simulink model "finalcode"  (R2020a)
settings: Solver=FixedStepDiscrete  StartTime=0.0  StopTime=1  FixedStep=0.0005  RelTol=1e-3  EnableMultiTasking=on
undefined symbols (not defined in the file): acc_calmax1, acc_calmax2, acc_calmin1, acc_calmin2, akemancanshu, angle_middle, bre, bre_calmax, bre_calmin, chasuniujvvvv_hou, chasuniujvvvv_qian, chasuuuu, ecucoder_acal, I_AN01_5K1, I_AN03_5V, I_AN04_5V, kd, kddd, ki, kiii, kp, kppp, leftmax, O_SW06_HS1A, P11111, P22222, PIDmodel, PPPP, rightmax, slip, slip_big, slip_little, slipmodel, T_add, T_del, tiaoshi, TTTTTyouren, vvvv, zhiling
libraries: ec5744lib x305, canmsglib x97, simulink x23
(part 3 of 11)

== system finalcode/无人TX/Toworkstation/toworkstation/toworkstation ==
  CAN Pack : canmsglib/CAN Pack  CANdbFile=C:\Users\Liu keliang\Desktop\HRT2023\HRT23赛季刘科良\CANdbc\toworkstation.dbc  MsgList=(none)  MsgName=toworkstation  MsgIDType=Standard (11-bit identifier)  MsgIdentifier=562  MsgLength=8  Remote=off  ApplyMinMax=off  BusOutput=off  SignalInfo={'youhou','0','16','LE','signed','Standard','0','1','0','-Inf','Inf';'youqian','16','16','LE','signed','Standard','0','1','0','-Inf','Inf';'zuohou','32','16','LE','signed','Standard','0','1','0','-Inf','Inf';'zuoqian','48','16','LE','signed','Standard','0','1','0','-Inf','Inf'}
      settings: SourceProductBaseCode=ME,XP,VN  DataFormat=CANdb specified signals
  CAN Pack1 : canmsglib/CAN Pack  CANdbFile=C:\Users\86155\Desktop\HRT2024\qkx\can\angle.dbc  MsgList=New_Message_3  MsgName=New_Message_3  MsgIDType=Standard (11-bit identifier)  MsgIdentifier=563  MsgLength=8  Remote=off  ApplyMinMax=off  BusOutput=off  SignalInfo={'actual_speed','48','16','LE','signed','Standard','0','1','0','-Inf','Inf';'bianmaqi','0','16','LE','signed','Standard','0','1','0','-Inf','Inf';'steer','16','16','LE','signed','Standard','0','1','0','-Inf','Inf';'target_speed','32','16','LE','unsigned','Standard','0','1','0','-Inf','Inf'}
      settings: SourceProductBaseCode=ME,XP,VN  DataFormat=CANdb specified signals
  CAN Pack2 : canmsglib/CAN Pack  CANdbFile=C:\Users\86155\Desktop\HRT2024\qkx\can\niujv.dbc  MsgList=New_Message_2  MsgName=New_Message_2  MsgIDType=Standard (11-bit identifier)  MsgIdentifier=561  MsgLength=8  Remote=off  ApplyMinMax=off  BusOutput=off  SignalInfo={'T_youhou','48','16','LE','signed','Standard','0','1','0','-Inf','Inf';'T_youqian','16','16','LE','signed','Standard','0','1','0','-Inf','Inf';'T_zuohou','32','16','LE','signed','Standard','0','1','0','-Inf','Inf';'T_zuoqian','0','16','LE','signed','Standard','0','1','0','-Inf','Inf'}
      settings: SourceProductBaseCode=ME,XP,VN  DataFormat=CANdb specified signals
  CANPackMessage : ec5744lib/RapidECU_U4B/04CANCommunication/CANPackMessage  datalength=8  sampletime=-1
      settings: SourceProductName=ECUCoder for MPC5744
  CANPackMessage1 : ec5744lib/RapidECU_U4B/04CANCommunication/CANPackMessage  datalength=8  sampletime=-1
      settings: SourceProductName=ECUCoder for MPC5744
  CANPackMessage2 : ec5744lib/RapidECU_U4B/04CANCommunication/CANPackMessage  datalength=8  sampletime=-1
      settings: SourceProductName=ECUCoder for MPC5744
  CANTransmit : ec5744lib/RapidECU_U4B/04CANCommunication/CANTransmit  canmodule=2  canbuffer=59  canmessageid=hex2dec('232')  canmessagetype=Standard(11-bit ID)  datalength=8  sampletime=-1
      settings: SourceProductName=ECUCoder for MPC5744
  CANTransmit1 : ec5744lib/RapidECU_U4B/04CANCommunication/CANTransmit  canmodule=2  canbuffer=63  canmessageid=hex2dec('233')  canmessagetype=Standard(11-bit ID)  datalength=8  sampletime=-1
      settings: SourceProductName=ECUCoder for MPC5744
  CANTransmit2 : ec5744lib/RapidECU_U4B/04CANCommunication/CANTransmit  canmodule=2  canbuffer=10  canmessageid=hex2dec('231')  canmessagetype=Standard(11-bit ID)  datalength=8  sampletime=-1
      settings: SourceProductName=ECUCoder for MPC5744
  Data Store Read : DataStoreRead  DataStoreName=er_v_lf
  Data Store Read1 : DataStoreRead  DataStoreName=er_v_rb
  Data Store Read10 : DataStoreRead  DataStoreName=torque_youhou
  Data Store Read11 : DataStoreRead  DataStoreName=energyr_youhou
  Data Store Read12 : DataStoreRead  DataStoreName=torque_zuoqian
  Data Store Read13 : DataStoreRead  DataStoreName=energyr_zuoqian
  Data Store Read14 : DataStoreRead  DataStoreName=workstation_steering
  Data Store Read15 : DataStoreRead  DataStoreName=V_guandao
  Data Store Read2 : DataStoreRead  DataStoreName=er_v_rf
  Data Store Read3 : DataStoreRead  DataStoreName=er_v_lb
  Data Store Read4 : DataStoreRead  DataStoreName=V_workstation
  Data Store Read5 : DataStoreRead  DataStoreName=steere
  Data Store Read6 : DataStoreRead  DataStoreName=torque_zuohou
  Data Store Read7 : DataStoreRead  DataStoreName=energyr_zuohou
  Data Store Read8 : DataStoreRead  DataStoreName=torque_youqian
  Data Store Read9 : DataStoreRead  DataStoreName=energyr_youqian
  Data Type Conversion : DataTypeConversion  OutDataTypeStr=uint8
  Data Type Conversion1 : DataTypeConversion  OutDataTypeStr=uint8
  Data Type Conversion2 : DataTypeConversion  OutDataTypeStr=uint8
  Gain{1..2,4..5} (4 alike) : Gain  Gain=1000
  MATLAB Function : MATLAB Function  TreatAsAtomicUnit=on
  MATLAB Function1 : MATLAB Function  TreatAsAtomicUnit=on
  MATLAB Function2 : MATLAB Function  TreatAsAtomicUnit=on
  MATLAB Function3 : MATLAB Function  TreatAsAtomicUnit=on
  MeaModule : ec5744lib/RapidECU_U4B/07Calibration/MeaModule  signal=T232
      settings: SourceProductName=ECUCoder for MPC5744
  MeaModule1 : ec5744lib/RapidECU_U4B/07Calibration/MeaModule  signal=T233
      settings: SourceProductName=ECUCoder for MPC5744
  Terminator : Terminator
  Terminator1 : Terminator
  Terminator2 : Terminator
  wires:
  CANPackMessage/1 -> Data Type Conversion/1
  CAN Pack/1 -> CANPackMessage/1
  CANTransmit/1 -> MeaModule/1
  MeaModule/1 -> Terminator/1
  Data Type Conversion/1 -> CANTransmit/1
  CANTransmit1/1 -> MeaModule1/1
  MeaModule1/1 -> Terminator1/1
  CANPackMessage1/1 -> Data Type Conversion1/1
  CAN Pack1/1 -> CANPackMessage1/1
  Data Type Conversion1/1 -> CANTransmit1/1
  Data Store Read14/1 -> Gain4/1
  Data Store Read5/1 -> Gain5/1
  Data Store Read1/1 -> CAN Pack/1
  Data Store Read2/1 -> CAN Pack/2
  Data Store Read3/1 -> CAN Pack/3
  Data Store Read/1 -> CAN Pack/4
  CANPackMessage2/1 -> Data Type Conversion2/1
  CANTransmit2/1 -> Terminator2/1
  CAN Pack2/1 -> CANPackMessage2/1
  Data Type Conversion2/1 -> CANTransmit2/1
  Data Store Read12/1 -> MATLAB Function/1(T)
  Data Store Read13/1 -> MATLAB Function/2(NT)
  MATLAB Function/1(y) -> CAN Pack2/4
  Data Store Read6/1 -> MATLAB Function1/1(T)
  Data Store Read7/1 -> MATLAB Function1/2(NT)
  MATLAB Function1/1(y) -> CAN Pack2/3
  Data Store Read8/1 -> MATLAB Function2/1(T)
  Data Store Read9/1 -> MATLAB Function2/2(NT)
  MATLAB Function2/1(y) -> CAN Pack2/2
  Data Store Read10/1 -> MATLAB Function3/1(T)
  Data Store Read11/1 -> MATLAB Function3/2(NT)
  MATLAB Function3/1(y) -> CAN Pack2/1
  Data Store Read4/1 -> Gain1/1
  Gain4/1 -> CAN Pack1/2
  Gain5/1 -> CAN Pack1/3
  Gain1/1 -> CAN Pack1/4
  Gain2/1 -> CAN Pack1/1
  Data Store Read15/1 -> Gain2/1

== system finalcode/Subsystem/Rx/283 285左前/Subsystem1/Subsystem ==
  ID : Inport
  msg : Inport  Port=2
  Enable : EnablePort
  CAN Pack : canmsglib/CAN Pack  Commented=on  CANdbFile=D:\desktop\enable.dbc  MsgList=(none)  MsgName=AMK_ActualValue1  MsgIDType=Standard (11-bit identifier)  MsgIdentifier=643  MsgLength=8  Remote=off  ApplyMinMax=off  BusOutput=off  SignalInfo={'AMK_ActualVelocity','16','16','LE','signed','Standard','0','1','0','0','65535';'AMK_MagnetizingCurrent','48','16','LE','signed','Standard','0','1','0','0','65535';'AMK_TorqueCurrent','32','16','LE','signed','Standard','0','1','0','0','65535';'AMK_bDcOn1','12','1','LE','unsigned','Standard','0','1','0','0','1';'AMK_bDerating1','15','1','LE','unsigned','Standard','0','1','0','0','1';'AMK_bError1','9','1','LE','unsigned','Standard','0','1','0','0','1';'AMK_bInverterOn1','14','1','LE','unsigned','Standard','0','1','0','0','1';'AMK_bQuitDcOn1','11','1','LE','unsigned','Standard','0','1','0','0','1';'AMK_bQuitInverterOn1','13','1','LE','unsigned','Standard','0','1','0','0','1';'AMK_bReserve1','0','8','LE','unsigned','Standard','0','1','0','0','255';'AMK_bSystemReady1','8','1','LE','unsigned','Standard','0','1','0','0','1';'AMK_bWarn1','10','1','LE','unsigned','Standard','0','1','0','0','1'}
      settings: SourceProductBaseCode=ME,XP,VN  DataFormat=CANdb specified signals
  CAN Unpack : canmsglib/CAN Unpack  CANdbFile=C:\Users\86155\Desktop\HRT2024\qkx\can\enable.dbc  MsgList=(none)  MsgName=AMK_ActualValue2  MsgIDType=Standard (11-bit identifier)  MsgIdentifier=645  MsgLength=8  SignalInfo={'AMK_ErrorInfo','32','16','LE','unsigned','Standard','0','1','0','0','65535';'AMK_TempIGBT','48','16','LE','signed','Standard','0','1','0','-32768','32767';'AMK_TempInverter','16','16','LE','signed','Standard','0','1','0','-32768','32767';'AMK_TempMotor','0','16','LE','signed','Standard','0','1','0','-32768','32767'}  IDPort=off  TimestampPort=off  ErrorPort=off  RemotePort=off  LengthPort=off  StatusPort=off  ApplyMinMax=off
      settings: SourceProductBaseCode=ME,XP,VN  DataFormat=CANdb specified signals
  CANPackMessage : ec5744lib/RapidECU_U4B/04CANCommunication/CANPackMessage  Commented=on  datalength=8  sampletime=-1
      settings: SourceProductName=ECUCoder for MPC5744
  CANUnPackMessage : ec5744lib/RapidECU_U4B/04CANCommunication/CANUnPackMessage  datalength=8  canmessagetype=Standard(11-bit ID)  sampletime=-1
      settings: SourceProductName=ECUCoder for MPC5744
  wires:
  msg/1 -> CANUnPackMessage/2
  CANUnPackMessage/1 -> CAN Unpack/1
  ID/1 -> CANUnPackMessage/1
  CANPackMessage/1 -> ?
  CAN Pack/1 -> CANPackMessage/1

== system finalcode/Subsystem/Rx/283 285左前/Subsystem2/Subsystem ==
  ID : Inport
  msg : Inport  Port=2
  Enable : EnablePort
  CAN Pack : canmsglib/CAN Pack  Commented=on  CANdbFile=D:\desktop\enable.dbc  MsgList=(none)  MsgName=AMK_ActualValue1  MsgIDType=Standard (11-bit identifier)  MsgIdentifier=643  MsgLength=8  Remote=off  ApplyMinMax=off  BusOutput=off  SignalInfo={'AMK_ActualVelocity','16','16','LE','signed','Standard','0','1','0','0','65535';'AMK_MagnetizingCurrent','48','16','LE','signed','Standard','0','1','0','0','65535';'AMK_TorqueCurrent','32','16','LE','signed','Standard','0','1','0','0','65535';'AMK_bDcOn1','12','1','LE','unsigned','Standard','0','1','0','0','1';'AMK_bDerating1','15','1','LE','unsigned','Standard','0','1','0','0','1';'AMK_bError1','9','1','LE','unsigned','Standard','0','1','0','0','1';'AMK_bInverterOn1','14','1','LE','unsigned','Standard','0','1','0','0','1';'AMK_bQuitDcOn1','11','1','LE','unsigned','Standard','0','1','0','0','1';'AMK_bQuitInverterOn1','13','1','LE','unsigned','Standard','0','1','0','0','1';'AMK_bReserve1','0','8','LE','unsigned','Standard','0','1','0','0','255';'AMK_bSystemReady1','8','1','LE','unsigned','Standard','0','1','0','0','1';'AMK_bWarn1','10','1','LE','unsigned','Standard','0','1','0','0','1'}
      settings: SourceProductBaseCode=ME,XP,VN  DataFormat=CANdb specified signals
  CAN Unpack : canmsglib/CAN Unpack  CANdbFile=C:\Users\86155\Desktop\HRT2024\qkx\can\enable.dbc  MsgList=(none)  MsgName=AMK_ActualValue1  MsgIDType=Standard (11-bit identifier)  MsgIdentifier=643  MsgLength=8  SignalInfo={'AMK_ActualVelocity','16','16','LE','signed','Standard','0','1','0','-32768','32767';'AMK_MagnetizingCurrent','48','16','LE','signed','Standard','0','1','0','-32768','32767';'AMK_TorqueCurrent','32','16','LE','signed','Standard','0','1','0','-32768','32767';'AMK_bDcOn1','12','1','LE','unsigned','Standard','0','1','0','0','1';'AMK_bDerating1','15','1','LE','unsigned','Standard','0','1','0','0','1';'AMK_bError1','9','1','LE','unsigned','Standard','0','1','0','0','1';'AMK_bInverterOn1','14','1','LE','unsigned','Standard','0','1','0','0','1';'AMK_bQuitDcOn1','11','1','LE','unsigned','Standard','0','1','0','0','1';'AMK_bQuitInverterOn1','13','1','LE','unsigned','Standard','0','1','0','0','1';'AMK_bReserve1','0','8','LE','unsigned','Standard','0','1','0','0','255';'AMK_bSystemReady1','8','1','LE','unsigned','Standard','0','1','0','0','1';'AMK_bWarn1','10','1','LE','unsigned','Standard','0','1','0','0','1'}  IDPort=off  TimestampPort=off  ErrorPort=off  RemotePort=off  LengthPort=off  StatusPort=off  ApplyMinMax=off
      settings: SourceProductBaseCode=ME,XP,VN  DataFormat=CANdb specified signals
  CANPackMessage : ec5744lib/RapidECU_U4B/04CANCommunication/CANPackMessage  Commented=on  datalength=8  sampletime=-1
      settings: SourceProductName=ECUCoder for MPC5744
  CANUnPackMessage : ec5744lib/RapidECU_U4B/04CANCommunication/CANUnPackMessage  datalength=8  canmessagetype=Standard(11-bit ID)  sampletime=-1
      settings: SourceProductName=ECUCoder for MPC5744
  Data Store Write : DataStoreWrite  DataStoreName=dianji_velcoity_zuoqian
  Data Store Write1 : DataStoreWrite  DataStoreName=er_v_lf
  Data Store Write2 : DataStoreWrite  DataStoreName=er_T_lf
  MATLAB Function : MATLAB Function  TreatAsAtomicUnit=on
  MeaModule : ec5744lib/RapidECU_U4B/07Calibration/MeaModule  signal=v_zuoqian
      settings: SourceProductName=ECUCoder for MPC5744
  wires:
  msg/1 -> CANUnPackMessage/2
  CANUnPackMessage/1 -> CAN Unpack/1
  ID/1 -> CANUnPackMessage/1
  CANPackMessage/1 -> ?
  CAN Unpack/1 -> Data Store Write1/1, MATLAB Function/1(u)
  MATLAB Function/1(y) -> MeaModule/1
  CAN Unpack/2 -> CAN Pack/2
  CAN Unpack/4 -> CAN Pack/5
  CAN Unpack/6 -> CAN Pack/8
  CAN Unpack/8 -> CAN Pack/11
  CAN Unpack/3 -> Data Store Write2/1
  MeaModule/1 -> Data Store Write/1

== system finalcode/Subsystem/Rx/284 286右前/Subsystem1/Subsystem ==
  ID : Inport
  msg : Inport  Port=2
  Enable : EnablePort
  CAN Pack : canmsglib/CAN Pack  Commented=on  CANdbFile=D:\desktop\enable.dbc  MsgList=(none)  MsgName=AMK_ActualValue1  MsgIDType=Standard (11-bit identifier)  MsgIdentifier=643  MsgLength=8  Remote=off  ApplyMinMax=off  BusOutput=off  SignalInfo={'AMK_ActualVelocity','16','16','LE','signed','Standard','0','1','0','0','65535';'AMK_MagnetizingCurrent','48','16','LE','signed','Standard','0','1','0','0','65535';'AMK_TorqueCurrent','32','16','LE','signed','Standard','0','1','0','0','65535';'AMK_bDcOn1','12','1','LE','unsigned','Standard','0','1','0','0','1';'AMK_bDerating1','15','1','LE','unsigned','Standard','0','1','0','0','1';'AMK_bError1','9','1','LE','unsigned','Standard','0','1','0','0','1';'AMK_bInverterOn1','14','1','LE','unsigned','Standard','0','1','0','0','1';'AMK_bQuitDcOn1','11','1','LE','unsigned','Standard','0','1','0','0','1';'AMK_bQuitInverterOn1','13','1','LE','unsigned','Standard','0','1','0','0','1';'AMK_bReserve1','0','8','LE','unsigned','Standard','0','1','0','0','255';'AMK_bSystemReady1','8','1','LE','unsigned','Standard','0','1','0','0','1';'AMK_bWarn1','10','1','LE','unsigned','Standard','0','1','0','0','1'}
      settings: SourceProductBaseCode=ME,XP,VN  DataFormat=CANdb specified signals
  CAN Unpack : canmsglib/CAN Unpack  CANdbFile=C:\Users\86155\Desktop\HRT2024\qkx\can\enable_youqian.dbc  MsgList=AMK_ActualValue2  MsgName=AMK_ActualValue2  MsgIDType=Standard (11-bit identifier)  MsgIdentifier=646  MsgLength=8  SignalInfo={'AMK_ErrorInfo','32','16','LE','unsigned','Standard','0','1','0','0','65535';'AMK_TempIGBT','48','16','LE','signed','Standard','0','1','0','-32768','32767';'AMK_TempInverter','16','16','LE','signed','Standard','0','1','0','-32768','32767';'AMK_TempMotor','0','16','LE','signed','Standard','0','1','0','-32768','32767'}  IDPort=off  TimestampPort=off  ErrorPort=off  RemotePort=off  LengthPort=off  StatusPort=off  ApplyMinMax=off
      settings: SourceProductBaseCode=ME,XP,VN  DataFormat=CANdb specified signals
  CANPackMessage : ec5744lib/RapidECU_U4B/04CANCommunication/CANPackMessage  Commented=on  datalength=8  sampletime=-1
      settings: SourceProductName=ECUCoder for MPC5744
  CANUnPackMessage : ec5744lib/RapidECU_U4B/04CANCommunication/CANUnPackMessage  datalength=8  canmessagetype=Standard(11-bit ID)  sampletime=-1
      settings: SourceProductName=ECUCoder for MPC5744
  wires:
  msg/1 -> CANUnPackMessage/2
  CANUnPackMessage/1 -> CAN Unpack/1
  ID/1 -> CANUnPackMessage/1
  CANPackMessage/1 -> ?
  CAN Pack/1 -> CANPackMessage/1

== system finalcode/Subsystem/Rx/284 286右前/Subsystem2/Subsystem ==
  ID : Inport
  msg : Inport  Port=2
  Enable : EnablePort
  CAN Pack : canmsglib/CAN Pack  Commented=on  CANdbFile=D:\desktop\enable.dbc  MsgList=(none)  MsgName=AMK_ActualValue1  MsgIDType=Standard (11-bit identifier)  MsgIdentifier=643  MsgLength=8  Remote=off  ApplyMinMax=off  BusOutput=off  SignalInfo={'AMK_ActualVelocity','16','16','LE','signed','Standard','0','1','0','0','65535';'AMK_MagnetizingCurrent','48','16','LE','signed','Standard','0','1','0','0','65535';'AMK_TorqueCurrent','32','16','LE','signed','Standard','0','1','0','0','65535';'AMK_bDcOn1','12','1','LE','unsigned','Standard','0','1','0','0','1';'AMK_bDerating1','15','1','LE','unsigned','Standard','0','1','0','0','1';'AMK_bError1','9','1','LE','unsigned','Standard','0','1','0','0','1';'AMK_bInverterOn1','14','1','LE','unsigned','Standard','0','1','0','0','1';'AMK_bQuitDcOn1','11','1','LE','unsigned','Standard','0','1','0','0','1';'AMK_bQuitInverterOn1','13','1','LE','unsigned','Standard','0','1','0','0','1';'AMK_bReserve1','0','8','LE','unsigned','Standard','0','1','0','0','255';'AMK_bSystemReady1','8','1','LE','unsigned','Standard','0','1','0','0','1';'AMK_bWarn1','10','1','LE','unsigned','Standard','0','1','0','0','1'}
      settings: SourceProductBaseCode=ME,XP,VN  DataFormat=CANdb specified signals
  CAN Unpack : canmsglib/CAN Unpack  CANdbFile=C:\Users\86155\Desktop\HRT2024\qkx\can\enable_youqian.dbc  MsgList=AMK_ActualValue1  MsgName=AMK_ActualValue1  MsgIDType=Standard (11-bit identifier)  MsgIdentifier=644  MsgLength=8  SignalInfo={'AMK_ActualVelocity','16','16','LE','signed','Standard','0','1','0','-32768','32767';'AMK_MagnetizingCurrent','48','16','LE','signed','Standard','0','1','0','-32768','32767';'AMK_TorqueCurrent','32','16','LE','signed','Standard','0','1','0','-32768','32767';'AMK_bDcOn1','12','1','LE','unsigned','Standard','0','1','0','0','1';'AMK_bDerating1','15','1','LE','unsigned','Standard','0','1','0','0','1';'AMK_bError1','9','1','LE','unsigned','Standard','0','1','0','0','1';'AMK_bInverterOn1','14','1','LE','unsigned','Standard','0','1','0','0','1';'AMK_bQuitDcOn1','11','1','LE','unsigned','Standard','0','1','0','0','1';'AMK_bQuitInverterOn1','13','1','LE','unsigned','Standard','0','1','0','0','1';'AMK_bReserve1','0','8','LE','unsigned','Standard','0','1','0','0','255';'AMK_bSystemReady1','8','1','LE','unsigned','Standard','0','1','0','0','1';'AMK_bWarn1','10','1','LE','unsigned','Standard','0','1','0','0','1'}  IDPort=off  TimestampPort=off  ErrorPort=off  RemotePort=off  LengthPort=off  StatusPort=off  ApplyMinMax=off
      settings: SourceProductBaseCode=ME,XP,VN  DataFormat=CANdb specified signals
  CANPackMessage : ec5744lib/RapidECU_U4B/04CANCommunication/CANPackMessage  Commented=on  datalength=8  sampletime=-1
      settings: SourceProductName=ECUCoder for MPC5744
  CANUnPackMessage : ec5744lib/RapidECU_U4B/04CANCommunication/CANUnPackMessage  datalength=8  canmessagetype=Standard(11-bit ID)  sampletime=-1
      settings: SourceProductName=ECUCoder for MPC5744
  Data Store Write : DataStoreWrite  DataStoreName=dianji_velcoity_youqian
  Data Store Write1 : DataStoreWrite  DataStoreName=er_v_rf
  Data Store Write2 : DataStoreWrite  DataStoreName=er_T_rf
  MATLAB Function : MATLAB Function  TreatAsAtomicUnit=on
  MeaModule : ec5744lib/RapidECU_U4B/07Calibration/MeaModule  signal=v_youqian
      settings: SourceProductName=ECUCoder for MPC5744
  wires:
  msg/1 -> CANUnPackMessage/2
  CANUnPackMessage/1 -> CAN Unpack/1
  ID/1 -> CANUnPackMessage/1
  CANPackMessage/1 -> ?
  CAN Pack/1 -> CANPackMessage/1
  CAN Unpack/1 -> Data Store Write1/1, MATLAB Function/1(u)
  MATLAB Function/1(y) -> MeaModule/1
  CAN Unpack/3 -> Data Store Write2/1
  MeaModule/1 -> Data Store Write/1

== system finalcode/Subsystem/Rx/287 289右后/Subsystem1/Subsystem ==
  ID : Inport
  msg : Inport  Port=2
  Enable : EnablePort
  CAN Pack : canmsglib/CAN Pack  Commented=on  CANdbFile=D:\desktop\enable.dbc  MsgList=(none)  MsgName=AMK_ActualValue1  MsgIDType=Standard (11-bit identifier)  MsgIdentifier=643  MsgLength=8  Remote=off  ApplyMinMax=off  BusOutput=off  SignalInfo={'AMK_ActualVelocity','16','16','LE','signed','Standard','0','1','0','0','65535';'AMK_MagnetizingCurrent','48','16','LE','signed','Standard','0','1','0','0','65535';'AMK_TorqueCurrent','32','16','LE','signed','Standard','0','1','0','0','65535';'AMK_bDcOn1','12','1','LE','unsigned','Standard','0','1','0','0','1';'AMK_bDerating1','15','1','LE','unsigned','Standard','0','1','0','0','1';'AMK_bError1','9','1','LE','unsigned','Standard','0','1','0','0','1';'AMK_bInverterOn1','14','1','LE','unsigned','Standard','0','1','0','0','1';'AMK_bQuitDcOn1','11','1','LE','unsigned','Standard','0','1','0','0','1';'AMK_bQuitInverterOn1','13','1','LE','unsigned','Standard','0','1','0','0','1';'AMK_bReserve1','0','8','LE','unsigned','Standard','0','1','0','0','255';'AMK_bSystemReady1','8','1','LE','unsigned','Standard','0','1','0','0','1';'AMK_bWarn1','10','1','LE','unsigned','Standard','0','1','0','0','1'}
      settings: SourceProductBaseCode=ME,XP,VN  DataFormat=CANdb specified signals
  CAN Unpack : canmsglib/CAN Unpack  CANdbFile=C:\Users\86155\Desktop\HRT2024\qkx\can\enable_youhou.dbc  MsgList=AMK_ActualValue2  MsgName=AMK_ActualValue2  MsgIDType=Standard (11-bit identifier)  MsgIdentifier=649  MsgLength=8  SignalInfo={'AMK_ErrorInfo','32','16','LE','unsigned','Standard','0','1','0','0','65535';'AMK_TempIGBT','48','16','LE','signed','Standard','0','1','0','-32768','32767';'AMK_TempInverter','16','16','LE','signed','Standard','0','1','0','-32768','32767';'AMK_TempMotor','0','16','LE','signed','Standard','0','1','0','-32768','32767'}  IDPort=off  TimestampPort=off  ErrorPort=off  RemotePort=off  LengthPort=off  StatusPort=off  ApplyMinMax=off
      settings: SourceProductBaseCode=ME,XP,VN  DataFormat=CANdb specified signals
  CANPackMessage : ec5744lib/RapidECU_U4B/04CANCommunication/CANPackMessage  Commented=on  datalength=8  sampletime=-1
      settings: SourceProductName=ECUCoder for MPC5744
  CANUnPackMessage : ec5744lib/RapidECU_U4B/04CANCommunication/CANUnPackMessage  datalength=8  canmessagetype=Standard(11-bit ID)  sampletime=-1
      settings: SourceProductName=ECUCoder for MPC5744
  wires:
  msg/1 -> CANUnPackMessage/2
  CANUnPackMessage/1 -> CAN Unpack/1
  ID/1 -> CANUnPackMessage/1
  CANPackMessage/1 -> ?
  CAN Pack/1 -> CANPackMessage/1

== system finalcode/Subsystem/Rx/287 289右后/Subsystem3/Subsystem ==
  ID : Inport
  msg : Inport  Port=2
  Enable : EnablePort
  CAN Pack : canmsglib/CAN Pack  Commented=on  CANdbFile=D:\desktop\enable.dbc  MsgList=(none)  MsgName=AMK_ActualValue1  MsgIDType=Standard (11-bit identifier)  MsgIdentifier=643  MsgLength=8  Remote=off  ApplyMinMax=off  BusOutput=off  SignalInfo={'AMK_ActualVelocity','16','16','LE','signed','Standard','0','1','0','0','65535';'AMK_MagnetizingCurrent','48','16','LE','signed','Standard','0','1','0','0','65535';'AMK_TorqueCurrent','32','16','LE','signed','Standard','0','1','0','0','65535';'AMK_bDcOn1','12','1','LE','unsigned','Standard','0','1','0','0','1';'AMK_bDerating1','15','1','LE','unsigned','Standard','0','1','0','0','1';'AMK_bError1','9','1','LE','unsigned','Standard','0','1','0','0','1';'AMK_bInverterOn1','14','1','LE','unsigned','Standard','0','1','0','0','1';'AMK_bQuitDcOn1','11','1','LE','unsigned','Standard','0','1','0','0','1';'AMK_bQuitInverterOn1','13','1','LE','unsigned','Standard','0','1','0','0','1';'AMK_bReserve1','0','8','LE','unsigned','Standard','0','1','0','0','255';'AMK_bSystemReady1','8','1','LE','unsigned','Standard','0','1','0','0','1';'AMK_bWarn1','10','1','LE','unsigned','Standard','0','1','0','0','1'}
      settings: SourceProductBaseCode=ME,XP,VN  DataFormat=CANdb specified signals
  CAN Unpack : canmsglib/CAN Unpack  CANdbFile=C:\Users\86155\Desktop\HRT2024\qkx\can\enable_youhou.dbc  MsgList=AMK_ActualValue1  MsgName=AMK_ActualValue1  MsgIDType=Standard (11-bit identifier)  MsgIdentifier=647  MsgLength=8  SignalInfo={'AMK_ActualVelocity','16','16','LE','signed','Standard','0','1','0','-32768','32767';'AMK_MagnetizingCurrent','48','16','LE','signed','Standard','0','1','0','-32768','32767';'AMK_TorqueCurrent','32','16','LE','signed','Standard','0','1','0','-32768','32767';'AMK_bDcOn1','12','1','LE','unsigned','Standard','0','1','0','0','1';'AMK_bDerating1','15','1','LE','unsigned','Standard','0','1','0','0','1';'AMK_bError1','9','1','LE','unsigned','Standard','0','1','0','0','1';'AMK_bInverterOn1','14','1','LE','unsigned','Standard','0','1','0','0','1';'AMK_bQuitDcOn1','11','1','LE','unsigned','Standard','0','1','0','0','1';'AMK_bQuitInverterOn1','13','1','LE','unsigned','Standard','0','1','0','0','1';'AMK_bReserve1','0','8','LE','unsigned','Standard','0','1','0','0','255';'AMK_bSystemReady1','8','1','LE','unsigned','Standard','0','1','0','0','1';'AMK_bWarn1','10','1','LE','unsigned','Standard','0','1','0','0','1'}  IDPort=off  TimestampPort=off  ErrorPort=off  RemotePort=off  LengthPort=off  StatusPort=off  ApplyMinMax=off
      settings: SourceProductBaseCode=ME,XP,VN  DataFormat=CANdb specified signals
  CANPackMessage : ec5744lib/RapidECU_U4B/04CANCommunication/CANPackMessage  Commented=on  datalength=8  sampletime=-1
      settings: SourceProductName=ECUCoder for MPC5744
  CANUnPackMessage : ec5744lib/RapidECU_U4B/04CANCommunication/CANUnPackMessage  datalength=8  canmessagetype=Standard(11-bit ID)  sampletime=-1
      settings: SourceProductName=ECUCoder for MPC5744
  Data Store Write : DataStoreWrite  DataStoreName=dianji_velcoity_youhou
  Data Store Write1 : DataStoreWrite  DataStoreName=er_v_rb
  Data Store Write2 : DataStoreWrite  DataStoreName=er_T_rb
  MATLAB Function : MATLAB Function  TreatAsAtomicUnit=on
  MeaModule : ec5744lib/RapidECU_U4B/07Calibration/MeaModule  signal=v_youhou
      settings: SourceProductName=ECUCoder for MPC5744
  wires:
  msg/1 -> CANUnPackMessage/2
  CANUnPackMessage/1 -> CAN Unpack/1
  ID/1 -> CANUnPackMessage/1
  CANPackMessage/1 -> ?
  CAN Pack/1 -> CANPackMessage/1
  MATLAB Function/1(y) -> MeaModule/1
  CAN Unpack/1 -> Data Store Write1/1, MATLAB Function/1(u)
  CAN Unpack/3 -> Data Store Write2/1
  MeaModule/1 -> Data Store Write/1

== system finalcode/Subsystem/Rx/288 290左后/Subsystem1/Subsystem ==
  ID : Inport
  msg : Inport  Port=2
  Enable : EnablePort
  CAN Pack : canmsglib/CAN Pack  Commented=on  CANdbFile=D:\desktop\enable.dbc  MsgList=(none)  MsgName=AMK_ActualValue1  MsgIDType=Standard (11-bit identifier)  MsgIdentifier=643  MsgLength=8  Remote=off  ApplyMinMax=off  BusOutput=off  SignalInfo={'AMK_ActualVelocity','16','16','LE','signed','Standard','0','1','0','0','65535';'AMK_MagnetizingCurrent','48','16','LE','signed','Standard','0','1','0','0','65535';'AMK_TorqueCurrent','32','16','LE','signed','Standard','0','1','0','0','65535';'AMK_bDcOn1','12','1','LE','unsigned','Standard','0','1','0','0','1';'AMK_bDerating1','15','1','LE','unsigned','Standard','0','1','0','0','1';'AMK_bError1','9','1','LE','unsigned','Standard','0','1','0','0','1';'AMK_bInverterOn1','14','1','LE','unsigned','Standard','0','1','0','0','1';'AMK_bQuitDcOn1','11','1','LE','unsigned','Standard','0','1','0','0','1';'AMK_bQuitInverterOn1','13','1','LE','unsigned','Standard','0','1','0','0','1';'AMK_bReserve1','0','8','LE','unsigned','Standard','0','1','0','0','255';'AMK_bSystemReady1','8','1','LE','unsigned','Standard','0','1','0','0','1';'AMK_bWarn1','10','1','LE','unsigned','Standard','0','1','0','0','1'}
      settings: SourceProductBaseCode=ME,XP,VN  DataFormat=CANdb specified signals
  CAN Unpack : canmsglib/CAN Unpack  CANdbFile=C:\Users\86155\Desktop\HRT2024\qkx\can\enabe_zuohou.dbc  MsgList=AMK_ActualValue2  MsgName=AMK_ActualValue2  MsgIDType=Standard (11-bit identifier)  MsgIdentifier=656  MsgLength=8  SignalInfo={'AMK_ErrorInfo','32','16','LE','unsigned','Standard','0','1','0','0','65535';'AMK_TempIGBT','48','16','LE','signed','Standard','0','1','0','-32768','32767';'AMK_TempInverter','16','16','LE','signed','Standard','0','1','0','-32768','32767';'AMK_TempMotor','0','16','LE','signed','Standard','0','1','0','-32768','32767'}  IDPort=off  TimestampPort=off  ErrorPort=off  RemotePort=off  LengthPort=off  StatusPort=off  ApplyMinMax=off
      settings: SourceProductBaseCode=ME,XP,VN  DataFormat=CANdb specified signals
  CANPackMessage : ec5744lib/RapidECU_U4B/04CANCommunication/CANPackMessage  Commented=on  datalength=8  sampletime=-1
      settings: SourceProductName=ECUCoder for MPC5744
  CANUnPackMessage : ec5744lib/RapidECU_U4B/04CANCommunication/CANUnPackMessage  datalength=8  canmessagetype=Standard(11-bit ID)  sampletime=-1
      settings: SourceProductName=ECUCoder for MPC5744
  wires:
  msg/1 -> CANUnPackMessage/2
  CANUnPackMessage/1 -> CAN Unpack/1
  ID/1 -> CANUnPackMessage/1
  CANPackMessage/1 -> ?
  CAN Pack/1 -> CANPackMessage/1

== system finalcode/Subsystem/Rx/288 290左后/Subsystem2/Subsystem ==
  ID : Inport
  msg : Inport  Port=2
  Enable : EnablePort
  CAN Pack : canmsglib/CAN Pack  Commented=on  CANdbFile=D:\desktop\enable.dbc  MsgList=(none)  MsgName=AMK_ActualValue1  MsgIDType=Standard (11-bit identifier)  MsgIdentifier=643  MsgLength=8  Remote=off  ApplyMinMax=off  BusOutput=off  SignalInfo={'AMK_ActualVelocity','16','16','LE','signed','Standard','0','1','0','0','65535';'AMK_MagnetizingCurrent','48','16','LE','signed','Standard','0','1','0','0','65535';'AMK_TorqueCurrent','32','16','LE','signed','Standard','0','1','0','0','65535';'AMK_bDcOn1','12','1','LE','unsigned','Standard','0','1','0','0','1';'AMK_bDerating1','15','1','LE','unsigned','Standard','0','1','0','0','1';'AMK_bError1','9','1','LE','unsigned','Standard','0','1','0','0','1';'AMK_bInverterOn1','14','1','LE','unsigned','Standard','0','1','0','0','1';'AMK_bQuitDcOn1','11','1','LE','unsigned','Standard','0','1','0','0','1';'AMK_bQuitInverterOn1','13','1','LE','unsigned','Standard','0','1','0','0','1';'AMK_bReserve1','0','8','LE','unsigned','Standard','0','1','0','0','255';'AMK_bSystemReady1','8','1','LE','unsigned','Standard','0','1','0','0','1';'AMK_bWarn1','10','1','LE','unsigned','Standard','0','1','0','0','1'}
      settings: SourceProductBaseCode=ME,XP,VN  DataFormat=CANdb specified signals
  CAN Unpack : canmsglib/CAN Unpack  CANdbFile=C:\Users\86155\Desktop\HRT2024\qkx\can\enabe_zuohou.dbc  MsgList=AMK_ActualValue1  MsgName=AMK_ActualValue1  MsgIDType=Standard (11-bit identifier)  MsgIdentifier=648  MsgLength=8  SignalInfo={'AMK_ActualVelocity','16','16','LE','signed','Standard','0','1','0','-32768','32767';'AMK_MagnetizingCurrent','48','16','LE','signed','Standard','0','1','0','-32768','32767';'AMK_TorqueCurrent','32','16','LE','signed','Standard','0','1','0','-32768','32767';'AMK_bDcOn1','12','1','LE','unsigned','Standard','0','1','0','0','1';'AMK_bDerating1','15','1','LE','unsigned','Standard','0','1','0','0','1';'AMK_bError1','9','1','LE','unsigned','Standard','0','1','0','0','1';'AMK_bInverterOn1','14','1','LE','unsigned','Standard','0','1','0','0','1';'AMK_bQuitDcOn1','11','1','LE','unsigned','Standard','0','1','0','0','1';'AMK_bQuitInverterOn1','13','1','LE','unsigned','Standard','0','1','0','0','1';'AMK_bReserve1','0','8','LE','unsigned','Standard','0','1','0','0','255';'AMK_bSystemReady1','8','1','LE','unsigned','Standard','0','1','0','0','1';'AMK_bWarn1','10','1','LE','unsigned','Standard','0','1','0','0','1'}  IDPort=off  TimestampPort=off  ErrorPort=off  RemotePort=off  LengthPort=off  StatusPort=off  ApplyMinMax=off
      settings: SourceProductBaseCode=ME,XP,VN  DataFormat=CANdb specified signals
  CANPackMessage : ec5744lib/RapidECU_U4B/04CANCommunication/CANPackMessage  Commented=on  datalength=8  sampletime=-1
      settings: SourceProductName=ECUCoder for MPC5744
  CANUnPackMessage : ec5744lib/RapidECU_U4B/04CANCommunication/CANUnPackMessage  datalength=8  canmessagetype=Standard(11-bit ID)  sampletime=-1
      settings: SourceProductName=ECUCoder for MPC5744
  Data Store Write : DataStoreWrite  DataStoreName=dianji_velcoity_zuohou
  Data Store Write1 : DataStoreWrite  DataStoreName=er_v_lb
  Data Store Write2 : DataStoreWrite  DataStoreName=er_T_lb
  MATLAB Function : MATLAB Function  TreatAsAtomicUnit=on
  MeaModule : ec5744lib/RapidECU_U4B/07Calibration/MeaModule  signal=v_zuohou
      settings: SourceProductName=ECUCoder for MPC5744
  wires:
  msg/1 -> CANUnPackMessage/2
  CANUnPackMessage/1 -> CAN Unpack/1
  ID/1 -> CANUnPackMessage/1
  CANPackMessage/1 -> ?
  CAN Pack/1 -> CANPackMessage/1
  CAN Unpack/1 -> Data Store Write1/1, MATLAB Function/1(u)
  CAN Unpack/3 -> Data Store Write2/1
  MATLAB Function/1(y) -> MeaModule/1
  MeaModule/1 -> Data Store Write/1
  CAN Unpack/2 -> CAN Pack/2
  CAN Unpack/4 -> CAN Pack/6
  CAN Unpack/5 -> CAN Pack/8
  CAN Unpack/6 -> CAN Pack/10
  CAN Unpack/7 -> CAN Pack/12

== system finalcode/Subsystem/Rx/ebs/Subsystem3/Subsystem ==
  ID : Inport
  msg : Inport  Port=2
  Enable : EnablePort
  CAN Pack : canmsglib/CAN Pack  Commented=on  CANdbFile=C:\Users\Liu keliang\Desktop\HRT2023\HRT23赛季刘科良\CANdbc\workstation.dbc  MsgList=(none)  MsgName=workstation  MsgIDType=Standard (11-bit identifier)  MsgIdentifier=32  MsgLength=5  Remote=off  ApplyMinMax=off  BusOutput=off  SignalInfo={'V','8','8','LE','unsigned','Standard','0','1','0','0','255';'V_Copy_1','16','8','LE','unsigned','Standard','0','1','0','0','255';'controlstart','4','1','LE','unsigned','Standard','0','1','0','-Inf','Inf';'status','0','4','LE','unsigned','Standard','0','1','0','0','15';'steering','24','8','LE','signed','Standard','0','1','0','-128','127';'steering_Copy_1','32','8','LE','signed','Standard','0','1','0','-128','127';'vfeedbackk','40','8','LE','unsigned','Standard','0','1','0','-Inf','Inf'}
      settings: SourceProductBaseCode=ME,XP,VN  DataFormat=CANdb specified signals
  CAN Unpack : canmsglib/CAN Unpack  CANdbFile=C:\Users\Liu keliang\Desktop\HRT2023\HRT23赛季刘科良\CANdbc\ebs.dbc  MsgList=(none)  MsgName=New_Message_1  MsgIDType=Standard (11-bit identifier)  MsgIdentifier=1026  MsgLength=8  SignalInfo={'youhou','48','16','LE','unsigned','Standard','0','1','0','-Inf','Inf';'youqian','16','16','LE','unsigned','Standard','0','1','0','-Inf','Inf';'zuohou','32','16','LE','unsigned','Standard','0','1','0','-Inf','Inf';'zuoqian','0','16','LE','unsigned','Standard','0','1','0','-Inf','Inf'}  IDPort=off  TimestampPort=off  ErrorPort=off  RemotePort=off  LengthPort=off  StatusPort=off  ApplyMinMax=off
      settings: SourceProductBaseCode=ME,XP,VN  DataFormat=CANdb specified signals
  CANPackMessage : ec5744lib/RapidECU_U4B/04CANCommunication/CANPackMessage  Commented=on  datalength=8  sampletime=-1
      settings: SourceProductName=ECUCoder for MPC5744
  CANUnPackMessage : ec5744lib/RapidECU_U4B/04CANCommunication/CANUnPackMessage  datalength=8  canmessagetype=Standard(11-bit ID)  sampletime=-1
      settings: SourceProductName=ECUCoder for MPC5744
  Data Store Write : DataStoreWrite  DataStoreName=oilyouhou
  Data Store Write1 : DataStoreWrite  DataStoreName=oilyouqian
  Data Store Write2 : DataStoreWrite  DataStoreName=oilzuohou
  Data Store Write3 : DataStoreWrite  DataStoreName=oilzuoqian
  wires:
  msg/1 -> CANUnPackMessage/2
  CANUnPackMessage/1 -> CAN Unpack/1
  ID/1 -> CANUnPackMessage/1
  CANPackMessage/1 -> ?
  CAN Pack/1 -> CANPackMessage/1
  CAN Unpack/2 -> Data Store Write1/1
  CAN Unpack/1 -> Data Store Write/1
  CAN Unpack/3 -> Data Store Write2/1
  CAN Unpack/4 -> Data Store Write3/1

== system finalcode/Subsystem/Rx/lcu——receive/Subsystem1/Subsystem ==
  ID : Inport
  msg : Inport  Port=2
  Enable : EnablePort
  CAN Pack : canmsglib/CAN Pack  Commented=on  CANdbFile=C:\Users\Liu keliang\Desktop\HRT2023\HRT23赛季刘科良\CANdbc\enzbled.dbc  MsgList=(none)  MsgName=ecu156  MsgIDType=Standard (11-bit identifier)  MsgIdentifier=342  MsgLength=8  Remote=off  ApplyMinMax=off  BusOutput=off  SignalInfo={'ASMS','3','1','LE','unsigned','Standard','0','1','0','-Inf','Inf';'enable','32','8','LE','unsigned','Standard','0','1','0','0','255';'error','16','8','LE','unsigned','Standard','0','1','0','0','255';'match_model','8','4','LE','unsigned','Standard','0','1','0','0','15';'matchmodel_shucai','24','3','LE','unsigned','Standard','0','1','0','0','6';'model_confirm','27','1','LE','unsigned','Standard','0','1','0','0','1';'res','40','3','LE','unsigned','Standard','0','1','0','-Inf','Inf';'ststus','0','3','LE','unsigned','Standard','0','1','0','0','7'}
      settings: SourceProductBaseCode=ME,XP,VN  DataFormat=CANdb specified signals
  CAN Unpack : canmsglib/CAN Unpack  CANdbFile=C:\Users\Liu keliang\Desktop\HRT2023\HRT23赛季刘科良\CANdbc\enzbled.dbc  MsgList=(none)  MsgName=ecu156  MsgIDType=Standard (11-bit identifier)  MsgIdentifier=342  MsgLength=8  SignalInfo={'ASMS','3','1','LE','unsigned','Standard','0','1','0','-Inf','Inf';'enable','32','8','LE','unsigned','Standard','0','1','0','0','255';'error','16','8','LE','unsigned','Standard','0','1','0','0','255';'match_model','8','4','LE','unsigned','Standard','0','1','0','0','15';'matchmodel_shucai','24','3','LE','unsigned','Standard','0','1','0','0','6';'model_confirm','27','1','LE','unsigned','Standard','0','1','0','0','1';'res','40','3','LE','unsigned','Standard','0','1','0','-Inf','Inf';'ststus','0','3','LE','unsigned','Standard','0','1','0','0','7'}  IDPort=off  TimestampPort=off  ErrorPort=off  RemotePort=off  LengthPort=off  StatusPort=off  ApplyMinMax=off
      settings: SourceProductBaseCode=ME,XP,VN  DataFormat=CANdb specified signals
  CANPackMessage : ec5744lib/RapidECU_U4B/04CANCommunication/CANPackMessage  Commented=on  datalength=8  sampletime=-1
      settings: SourceProductName=ECUCoder for MPC5744
  CANUnPackMessage : ec5744lib/RapidECU_U4B/04CANCommunication/CANUnPackMessage  datalength=8  canmessagetype=Standard(11-bit ID)  sampletime=-1
      settings: SourceProductName=ECUCoder for MPC5744
  Data Store Write : DataStoreWrite  DataStoreName=match_model
  Data Store Write1 : DataStoreWrite  DataStoreName=status
  Data Store Write2 : DataStoreWrite  DataStoreName=nengpao
  MATLAB Function : MATLAB Function  Commented=on  TreatAsAtomicUnit=on
  MATLAB Function1 : MATLAB Function  TreatAsAtomicUnit=on
  MATLAB Function2 : MATLAB Function  TreatAsAtomicUnit=on
  MeaModule8 : ec5744lib/RapidECU_U4B/07Calibration/MeaModule  signal=enable
      settings: SourceProductName=ECUCoder for MPC5744
  缓停 : DataStoreWrite  DataStoreName=huanting
  CAN_msg_enable : Outport
  wires:
  msg/1 -> CANUnPackMessage/2
  CANUnPackMessage/1 -> CAN Unpack/1
  ID/1 -> CANUnPackMessage/1
  CAN Pack/1 -> CANPackMessage/1
  CAN Unpack/3 -> CAN Pack/3
  CAN Unpack/4 -> Data Store Write/1, CAN Pack/4
  CAN Unpack/5 -> CAN Pack/5
  CAN Unpack/6 -> CAN Pack/6
  MeaModule8/1 -> CAN_msg_enable/1
  CAN Unpack/1 -> CAN Pack/1
  CAN Unpack/2 -> MeaModule8/1, CAN Pack/2
  MATLAB Function1/1(y) -> 缓停/1
  MATLAB Function2/1(y) -> Data Store Write2/1
  CAN Unpack/8 -> MATLAB Function1/1(u), MATLAB Function2/1(u), Data Store Write1/1

== system finalcode/Subsystem/Rx/shucai—receive/Subsystem1/Subsystem ==
  ID : Inport
  msg : Inport  Port=2
  Enable : EnablePort
  CAN Unpack : canmsglib/CAN Unpack  CANdbFile=C:\Users\18137\Desktop\0429\HRT_23E.dbc  MsgList=(none)  MsgName=shucai_xyz  MsgIDType=Standard (11-bit identifier)  MsgIdentifier=18  MsgLength=8  SignalInfo={'shucai_ax','16','16','LE','signed','Standard','0','1','0','-32768','32768';'shucai_ay','32','16','LE','signed','Standard','0','1','0','-32768','32767';'shucai_az','48','16','LE','signed','Standard','0','1','0','-32768','32767'}  IDPort=off  TimestampPort=off  ErrorPort=off  RemotePort=off  LengthPort=off  StatusPort=off  ApplyMinMax=off
      settings: SourceProductBaseCode=ME,XP,VN  DataFormat=CANdb specified signals
  CANUnPackMessage : ec5744lib/RapidECU_U4B/04CANCommunication/CANUnPackMessage  datalength=8  canmessagetype=Standard(11-bit ID)  sampletime=-1
      settings: SourceProductName=ECUCoder for MPC5744
  Data Store Write : DataStoreWrite  DataStoreName=shucai_ax
  Data Store Write1 : DataStoreWrite  DataStoreName=shucai_ay
  Data Store Write2 : DataStoreWrite  DataStoreName=shucai_az
  MATLAB Function : MATLAB Function  TreatAsAtomicUnit=on
  wires:
  msg/1 -> CANUnPackMessage/2
  CANUnPackMessage/1 -> CAN Unpack/1
  ID/1 -> CANUnPackMessage/1
  CAN Unpack/2 -> MATLAB Function/2(y)
  CAN Unpack/1 -> MATLAB Function/1(x)
  CAN Unpack/3 -> MATLAB Function/3(z)
  MATLAB Function/2(ay) -> Data Store Write1/1
  MATLAB Function/1(ax) -> Data Store Write/1
  MATLAB Function/3(az) -> Data Store Write2/1

== system finalcode/Subsystem/Rx/工作站/Subsystem1/Subsystem1 ==
  ID : Inport
  msg : Inport  Port=2
  Enable : EnablePort
  Subsystem : Subsystem
  wires:
  ID/1 -> Subsystem/1(ID)
  msg/1 -> Subsystem/2(msg)

== system finalcode/Subsystem/Rx/工作站/Subsystem3/Subsystem ==
  ID : Inport
  msg : Inport  Port=2
  Enable : EnablePort
  Add : Sum
  Add1 : Sum
  Add2 : Sum
  CAN Pack : canmsglib/CAN Pack  Commented=on  CANdbFile=C:\Users\Liu keliang\Desktop\HRT2023\HRT23赛季刘科良\CANdbc\workstation.dbc  MsgList=(none)  MsgName=workstation  MsgIDType=Standard (11-bit identifier)  MsgIdentifier=32  MsgLength=5  Remote=off  ApplyMinMax=off  BusOutput=off  SignalInfo={'V','8','8','LE','unsigned','Standard','0','1','0','0','255';'V_Copy_1','16','8','LE','unsigned','Standard','0','1','0','0','255';'controlstart','4','1','LE','unsigned','Standard','0','1','0','-Inf','Inf';'status','0','4','LE','unsigned','Standard','0','1','0','0','15';'steering','24','8','LE','signed','Standard','0','1','0','-128','127';'steering_Copy_1','32','8','LE','signed','Standard','0','1','0','-128','127';'vfeedbackk','40','8','LE','unsigned','Standard','0','1','0','-Inf','Inf'}
      settings: SourceProductBaseCode=ME,XP,VN  DataFormat=CANdb specified signals
  CAN Unpack : canmsglib/CAN Unpack  CANdbFile=C:\Users\86155\Desktop\HRT2024\qkx\can\workstation.dbc  MsgList=workstation  MsgName=workstation  MsgIDType=Standard (11-bit identifier)  MsgIdentifier=32  MsgLength=7  SignalInfo={'V','8','8','LE','unsigned','Standard','0','1','0','0','255';'V_Copy_1','16','8','LE','unsigned','Standard','0','1','0','0','255';'V_actual','40','8','LE','signed','Standard','0','1','0','-Inf','Inf';'V_actual_Copy','48','8','LE','signed','Standard','0','1','0','-Inf','Inf';'status','0','4','LE','unsigned','Standard','0','1','0','0','15';'steering','24','8','LE','signed','Standard','0','1','0','-128','127';'steering_Copy_1','32','8','LE','signed','Standard','0','1','0','-128','127'}  IDPort=off  TimestampPort=off  ErrorPort=off  RemotePort=off  LengthPort=off  StatusPort=off  ApplyMinMax=off
      settings: SourceProductBaseCode=ME,XP,VN  DataFormat=CANdb specified signals
  CANPackMessage : ec5744lib/RapidECU_U4B/04CANCommunication/CANPackMessage  Commented=on  datalength=8  sampletime=-1
      settings: SourceProductName=ECUCoder for MPC5744
  CANUnPackMessage : ec5744lib/RapidECU_U4B/04CANCommunication/CANUnPackMessage  datalength=7  canmessagetype=Standard(11-bit ID)  sampletime=-1
      settings: SourceProductName=ECUCoder for MPC5744
  Data Store Read1 : DataStoreRead  DataStoreName=nengpao
  Data Store Read3 : DataStoreRead  DataStoreName=match_model
  Data Store Write : DataStoreWrite  DataStoreName=V_workstation
  Data Store Write1 : DataStoreWrite  DataStoreName=workstation_status
  Data Store Write2 : DataStoreWrite  DataStoreName=workstation_steering
  Data Store Write3 : DataStoreWrite  DataStoreName=V_guandao
  Gain : Gain  Gain=-1
  MATLAB Function : MATLAB Function  TreatAsAtomicUnit=on
  MATLAB Function1 : MATLAB Function  TreatAsAtomicUnit=on
  MATLAB Function2 : MATLAB Function  TreatAsAtomicUnit=on
  MATLAB Function3 : MATLAB Function  TreatAsAtomicUnit=on
  MATLAB Function4 : MATLAB Function  TreatAsAtomicUnit=on
  MATLAB Function5 : MATLAB Function  Commented=on  TreatAsAtomicUnit=on
  MATLAB Function6 : MATLAB Function  Commented=on  TreatAsAtomicUnit=on
  MATLAB Function7 : MATLAB Function  TreatAsAtomicUnit=on
  MATLAB Function8 : MATLAB Function  TreatAsAtomicUnit=on
  MeaModule2 : ec5744lib/RapidECU_U4B/07Calibration/MeaModule  signal=steer_workstation
      settings: SourceProductName=ECUCoder for MPC5744
  Subsystem : Subsystem
  wires:
  msg/1 -> CANUnPackMessage/2
  CANUnPackMessage/1 -> CAN Unpack/1
  ID/1 -> CANUnPackMessage/1
  CANPackMessage/1 -> ?
  CAN Pack/1 -> CANPackMessage/1
  CAN Unpack/1 -> MATLAB Function/1(u)
  Add1/1 -> Gain/1
  MATLAB Function/1(y) -> Add/1
  MATLAB Function2/1(y) -> Add/2
  MATLAB Function3/1(y) -> Add1/2
  MATLAB Function1/1(y) -> Add1/1
  MATLAB Function4/1(y) -> Data Store Write/1
  Data Store Read1/1 -> MATLAB Function4/2(nengbunengpao)
  Add/1 -> MATLAB Function4/1(u)
  Data Store Read3/1 -> MATLAB Function4/3(model)
  CAN Unpack/2 -> MATLAB Function2/1(u)
  Subsystem/1(Out1) -> MATLAB Function8/2(CANOK_20), MATLAB Function7/2(CANOK_20), MATLAB Function3/3(CANOK_20), MATLAB Function1/2(CANOK_20), MATLAB Function2/2(CANOK_20), MATLAB Function/2(CANOK_20)
  MeaModule2/1 -> Data Store Write2/1
  CAN Unpack/7 -> MATLAB Function3/2(u)
  CAN Unpack/6 -> MATLAB Function3/1(steer), MATLAB Function1/1(u)
  CAN Unpack/5 -> Data Store Write1/1
  MATLAB Function7/1(y) -> Add2/1
  MATLAB Function8/1(y) -> Add2/2
  CAN Unpack/3 -> MATLAB Function7/1(u)
  CAN Unpack/4 -> MATLAB Function8/1(u)
  Add2/1 -> Data Store Write3/1
  Gain/1 -> MeaModule2/1

== system finalcode/Subsystem/Rx/惯导/Subsystem1/Subsystem ==
  ID : Inport
  msg : Inport  Port=2
  Enable : EnablePort
  CAN Pack : canmsglib/CAN Pack  Commented=on  CANdbFile=D:\desktop\enable.dbc  MsgList=(none)  MsgName=AMK_ActualValue1  MsgIDType=Standard (11-bit identifier)  MsgIdentifier=643  MsgLength=8  Remote=off  ApplyMinMax=off  BusOutput=off  SignalInfo={'AMK_ActualVelocity','16','16','LE','signed','Standard','0','1','0','0','65535';'AMK_MagnetizingCurrent','48','16','LE','signed','Standard','0','1','0','0','65535';'AMK_TorqueCurrent','32','16','LE','signed','Standard','0','1','0','0','65535';'AMK_bDcOn1','12','1','LE','unsigned','Standard','0','1','0','0','1';'AMK_bDerating1','15','1','LE','unsigned','Standard','0','1','0','0','1';'AMK_bError1','9','1','LE','unsigned','Standard','0','1','0','0','1';'AMK_bInverterOn1','14','1','LE','unsigned','Standard','0','1','0','0','1';'AMK_bQuitDcOn1','11','1','LE','unsigned','Standard','0','1','0','0','1';'AMK_bQuitInverterOn1','13','1','LE','unsigned','Standard','0','1','0','0','1';'AMK_bReserve1','0','8','LE','unsigned','Standard','0','1','0','0','255';'AMK_bSystemReady1','8','1','LE','unsigned','Standard','0','1','0','0','1';'AMK_bWarn1','10','1','LE','unsigned','Standard','0','1','0','0','1'}
      settings: SourceProductBaseCode=ME,XP,VN  DataFormat=CANdb specified signals
  CAN Unpack : canmsglib/CAN Unpack  CANdbFile=C:\Users\Liu keliang\Desktop\HRT2023\HRT23赛季刘科良\CANdbc\homework1.dbc  MsgList=(none)  MsgName=INS_HeadingPitchRoll  MsgIDType=Standard (11-bit identifier)  MsgIdentifier=1282  MsgLength=7  SignalInfo={'INS_HeadingAngle','48','16','BE','unsigned','Standard','0','0.010986','-360','-360','360';'INS_PitchAngle','16','16','BE','unsigned','Standard','0','0.010986','-360','-360','360';'INS_RollAngle','32','16','BE','unsigned','Standard','0','0.010986','-360','-360','360'}  IDPort=off  TimestampPort=off  ErrorPort=off  RemotePort=off  LengthPort=off  StatusPort=off  ApplyMinMax=off
      settings: SourceProductBaseCode=ME,XP,VN  DataFormat=CANdb specified signals
  CANPackMessage : ec5744lib/RapidECU_U4B/04CANCommunication/CANPackMessage  Commented=on  datalength=8  sampletime=-1
      settings: SourceProductName=ECUCoder for MPC5744
  CANUnPackMessage : ec5744lib/RapidECU_U4B/04CANCommunication/CANUnPackMessage  datalength=7  canmessagetype=Standard(11-bit ID)  sampletime=-1
      settings: SourceProductName=ECUCoder for MPC5744
  wires:
  msg/1 -> CANUnPackMessage/2
  CANUnPackMessage/1 -> CAN Unpack/1
  ID/1 -> CANUnPackMessage/1
  CAN Pack/1 -> CANPackMessage/1
